simulink model "sigma_delta_1er_ordre"  (R2024a)
settings: Solver=ode3  StartTime=0.0  StopTime=1-ts  FixedStep=ts  RelTol=1e-3  EnableMultiTasking=on
values from neighbouring files (symbols this model uses):
  fck = 1000000    [main_sigma_delta.m]
  noise_laplace = 10^-10    (= 1e-10)    [main_sigma_delta.m]
  tau = 1/(2*pi*fc)    (= 0.0159154943092)    [main_sigma_delta.m]
  ts = 0.000001    (= 1e-06)    [main_sigma_delta.m]
libraries: simulink x1
settings Model: Creator=mailly  LastModifiedBy=diogo.klafke-ogochi
settings SolverCC: AlgebraicLoopSolver=TrustRegion
settings DataIOCC: LimitDataPoints=on  SaveFormat=Array  SignalLoggingSaveFormat=ModelDataLogs  ReturnWorkspaceOutputs=off
settings OptimizationCC: InitFltsAndDblsToZero=on  LifeSpan=inf
settings DebuggingCC: SaveWithParameterizedLinksMsg=none  UnderspecifiedInitializationDetection=Classic  MergeDetectMultiDrivingBlocksExec=none  SignalResolutionControl=TryResolveAllWithWarning  SolverPrmCheckMsg=warning  MultiTaskDSMMsg=warning  MultiTaskCondExecSysMsg=none  FcnCallInpInsideContextMsg=warning  UnconnectedInputMsg=warning  UnconnectedOutputMsg=warning  UnconnectedLineMsg=warning  AllowSymbolicDim=off  SFUnexpectedBacktrackingDiag=warning  SFNoUnconditionalDefaultTransitionDiag=warning  SFExecutionAtInitializationDiag=none  ArithmeticOperatorsInVariantConditions=warning
settings HardwareCC: ProdBitPerPointer=32  ProdBitPerSizeT=32  ProdBitPerPtrDiffT=32  ProdLargestAtomicFloat=None  ProdIntDivRoundTo=Undefined  ProdEndianess=Unspecified  ProdWordSize=32  ProdHWDeviceType=32-bit Generic
settings ModelReferenceCC: EnableRefExpFcnMdlSchedulingChecks=on  PropagateSignalLabelsOutOfModel=off
settings SFSimCC: SimUseLocalCustomCode=off  CustomCodeUndefinedFunction=UseInterfaceOnly
settings RTWCC: RTWUseLocalCustomCode=off  GPUComputeCapability=3.5
settings CodeAppCC: StateflowObjectComments=on
settings GRTTargetCC: TargetFcnLib=ansi_tfl_tmw.mat  TargetLangStandard=C89/C90 (ANSI)  CombineOutputUpdateFcns=off  GRTInterface=on
settings ConfigComp: CovMetricSettings=dw  CovSaveCumulativeToWorkspaceVar=on  CovSaveSingleToWorkspaceVar=on  CovExternalEMLEnable=off

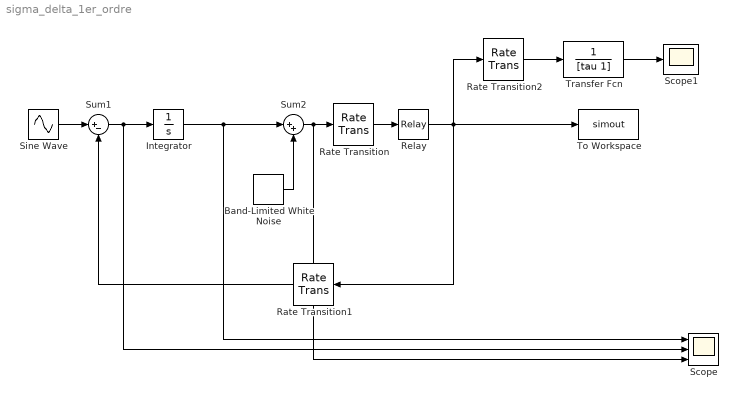
== system sigma_delta_1er_ordre ==
  Band-Limited White Noise : simulink/Sources/Band-Limited White Noise  Cov=[noise_laplace]  Ts=ts  seed=[23341]
  Integrator : Integrator
  Rate Transition : RateTransition
  Rate Transition1 : RateTransition
  Rate Transition2 : RateTransition
  Relay : Relay  OnSwitchValue=0  OffSwitchValue=0  OffOutputValue=-1  SampleTime=1/fck
  Scope : Scope  NumInputPorts=3
  Scope1 : Scope
  Sine Wave : Sin  Amplitude=0.5  Frequency=2*pi*10  SampleTime=ts
  Sum1 : Sum  Inputs=|+-
  Sum2 : Sum  Inputs=|++
  To Workspace : ToWorkspace  VariableName=simout  SampleTime=1/fck
      settings: MaxDataPoints=fck
  Transfer Fcn : TransferFcn  Denominator=[tau 1]
  wires:
  Sine Wave/1 -> Sum1/1
  Sum1/1 -> Scope/2, Integrator/1
  Relay/1 -> To Workspace/1, Rate Transition1/1, Rate Transition2/1
  Rate Transition1/1 -> Sum1/2
  Band-Limited White Noise/1 -> Sum2/2
  Sum2/1 -> Rate Transition/1, Scope/3
  Rate Transition/1 -> Relay/1
  Transfer Fcn/1 -> Scope1/1
  Rate Transition2/1 -> Transfer Fcn/1
  Integrator/1 -> Sum2/1, Scope/1
